simulink model "testFT_sensor"  (Simulink 8.7)
settings: Solver=FixedStepDiscrete  StartTime=0.0  StopTime=inf  FixedStep=ts  RelTol=1e-3
values from neighbouring files (symbols this model uses):
  gazebo_H_base = [Rfoot posFoot; 0 0 0 1]    [initTorqueBalancing.m]    (also in initTorqueBalancingPC.m)
  gazebo_H_chair = [eye(3),[0;0;0.165]; 0 0 0 1]    [initTorqueBalancing.m]    (also in initTorqueBalancingPC.m)
  link2_corr = -9.8    [initTorqueBalancing.m]    (also in initTorqueBalancingPC.m)
undefined symbols (not defined in the file or in its folder): CONFIG, WBT_robotName
libraries: WBToolboxLibrary x13
settings Model: Creator=DanielePucci  LastModifiedBy=gnava
settings DataIOCC: LimitDataPoints=off  SaveFormat=Dataset
settings DebuggingCC: UnderspecifiedInitializationDetection=Simplified  MergeDetectMultiDrivingBlocksExec=error
settings HardwareCC: ProdBitPerPointer=64  ProdLargestAtomicFloat=Float  ProdIntDivRoundTo=Zero  ProdEndianess=LittleEndian  ProdWordSize=64  ProdHWDeviceType=Intel->x86-64 (Windows64)
settings ModelReferenceCC: PropagateSignalLabelsOutOfModel=on
settings ConfigComp: CovModelRefEnable=off

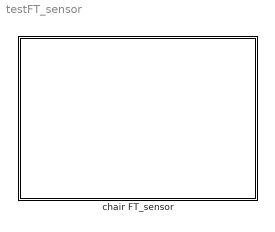
== system testFT_sensor ==
  chair FT_sensor : Subsystem

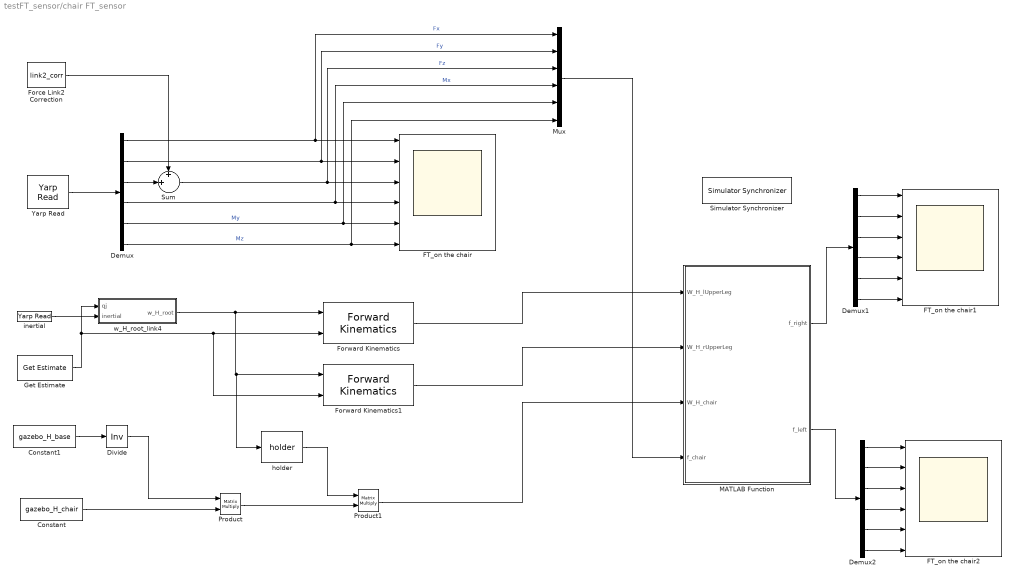
== system testFT_sensor/chair FT_sensor ==
  Constant : Constant  Value=gazebo_H_chair
  Constant1 : Constant  Value=gazebo_H_base
  Demux : Demux  Outputs=6
  Demux1 : Demux  Outputs=6
  Demux2 : Demux  Outputs=6
  Divide : Product  Inputs=/  Multiplication=Matrix(*)
  FT_on the chair : Scope  NumInputPorts=6
  FT_on the chair1 : Scope  NumInputPorts=6
  FT_on the chair2 : Scope  NumInputPorts=6
  Force Link2 Correction : Constant  Value=link2_corr
  Forward Kinematics : WBToolboxLibrary/wholeBodyModel/Kinematics/Forward Kinematics  frameName='l_upper_leg'  robotName=WBT_robotName  localName=WBT_modelName  wbiFile=WBT_wbiFilename  wbiList=WBT_wbiList
  Forward Kinematics1 : WBToolboxLibrary/wholeBodyModel/Kinematics/Forward Kinematics  frameName='r_upper_leg'  robotName=WBT_robotName  localName=WBT_modelName  wbiFile=WBT_wbiFilename  wbiList=WBT_wbiList
  Get Estimate : WBToolboxLibrary/wholeBodyStates/Get Estimate  estimateType=Joints Position  robotName=WBT_robotName  localName=WBT_modelName  wbiFile=WBT_wbiFilename  wbiList=WBT_wbiList
  MATLAB Function : MATLAB Function  TreatAsAtomicUnit=on
  Mux : Mux  Inputs=6
  Product : Product  Multiplication=Matrix(*)
  Product1 : Product  Multiplication=Matrix(*)
  Simulator Synchronizer : WBToolboxLibrary/Utilities/Simulator Synchronizer  period=ts  serverPortName='/clock/rpc'  clientPortName='/WBT_synchronizer/rpc:o'
  Sum : Sum  Inputs=+|+||
  Yarp Read : WBToolboxLibrary/Utilities/Yarp Read  portName=PORTS.WBDT_CHAIR  signalSize=6  blocking=off  timestamp=off  autoconnect=on  errorOnConnection=on
  "holder " : WBToolboxLibrary/Utilities/holder 
  inertial : WBToolboxLibrary/Utilities/Yarp Read  portName=PORTS.IMU  signalSize=12  blocking=off  timestamp=off  autoconnect=on  errorOnConnection=on
  w_H_root_link4 : Subsystem  mask{link_name='l_sole'}
      mask prompts: link_name "link name"
      mask help:
      | This block evaluates the homogeneous transformation between the world and the root link, i.e. ^wH_b. It assumes that the link specified by the variable 'link_name' has a constant position
      | w.r.t. an inertial frame, but it can rotate arbitrarily. This rotation is retrived from the IMU sensor.
      mask Display:
      | str = strrep(link_name, '_','\_');
      | port_label('output',1,['{}^{',str '}H_{root}'],'texmode','on')
      | clear str;
      | 
      | port_label('input',1,'q_j','texmode','on')
      | 
      | port_label('input',2,'inertial','texmode','on')
  wires:
  Demux1/4 -> FT_on the chair1/4
  Constant1/1 -> Divide/1
  MATLAB Function/2(f_left) -> Demux2/1
  MATLAB Function/1(f_right) -> Demux1/1
  Product/1 -> Product1/2
  Demux1/5 -> FT_on the chair1/5
  Demux1/6 -> FT_on the chair1/6
  Demux1/2 -> FT_on the chair1/2
  Forward Kinematics/1 -> MATLAB Function/1(W_H_lUpperLeg)
  "holder "/1 -> Product1/1
  Demux2/4 -> FT_on the chair2/4
  w_H_root_link4/1(w_H_root) -> "holder "/1, Forward Kinematics1/1, Forward Kinematics/1
  Demux1/1 -> FT_on the chair1/1
  Forward Kinematics1/1 -> MATLAB Function/2(W_H_rUpperLeg)
  Mux/1 -> MATLAB Function/4(f_chair)
  Product1/1 -> MATLAB Function/3(W_H_chair)
  Divide/1 -> Product/1
  Constant/1 -> Product/2
  Demux1/3 -> FT_on the chair1/3
  Demux2/2 -> FT_on the chair2/2
  Demux2/5 -> FT_on the chair2/5
  Demux2/3 -> FT_on the chair2/3
  Demux2/6 -> FT_on the chair2/6
  Demux2/1 -> FT_on the chair2/1
  Yarp Read/1 -> Demux/1
  Demux/1 -> FT_on the chair/1, Mux/1  "Fx"
  Demux/2 -> FT_on the chair/2, Mux/2  "Fy"
  Demux/5 -> FT_on the chair/5, Mux/5  "My"
  Demux/4 -> FT_on the chair/4, Mux/4  "Mx"
  Demux/6 -> FT_on the chair/6, Mux/6  "Mz"
  Force Link2 Correction/1 -> Sum/1
  Demux/3 -> Sum/2
  Sum/1 -> FT_on the chair/3, Mux/3  "Fz"
  Get Estimate/1 -> Forward Kinematics1/2, Forward Kinematics/2, w_H_root_link4/1(qj)
  inertial/1 -> w_H_root_link4/2(inertial)

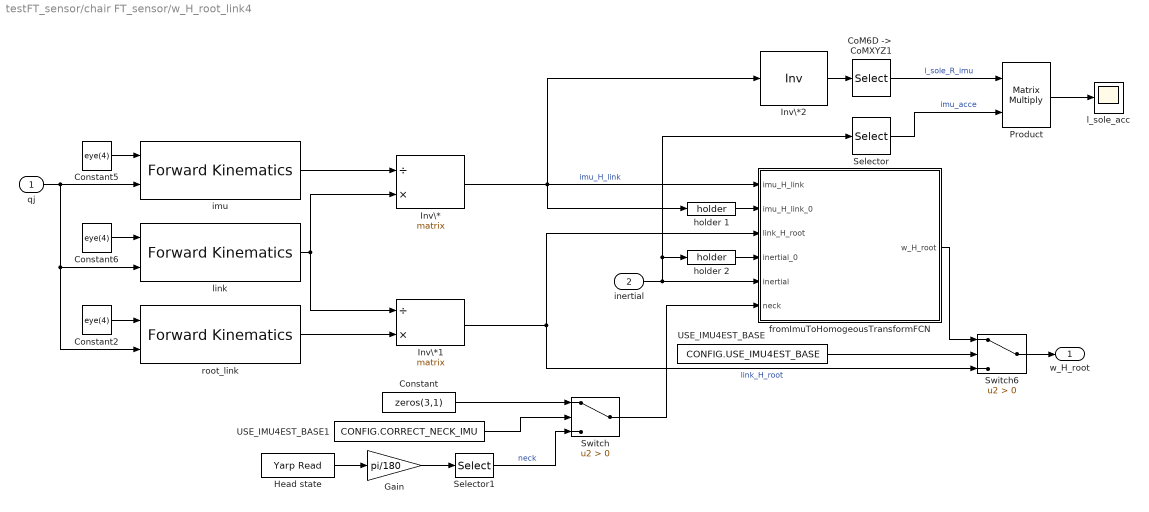
== system testFT_sensor/chair FT_sensor/w_H_root_link4 ==
  qj : Inport
  inertial : Inport  Port=2
  "CoM6D ->  CoMXYZ1" : Selector  NumberOfDimensions=2  InputPortWidth=7  IndexOptions=Index vector (dialog),Index vector (dialog)  Indices=[1 2 3],[1 2 3]  OutputSizes=1,1
  Constant : Constant  Value=zeros(3,1)
  Constant2 : Constant  Value=eye(4)
  Constant5 : Constant  Value=eye(4)
  Constant6 : Constant  Value=eye(4)
  Gain : Gain  Gain=pi/180
  Head state : WBToolboxLibrary/Utilities/Yarp Read  portName=[WBT_robotName, '/head/state:o']  signalSize=6  blocking=off  timestamp=off  autoconnect=on  errorOnConnection=off
  Inv\* : Product  Inputs=/*  Multiplication=Matrix(*)
  Inv\*1 : Product  Inputs=/*  Multiplication=Matrix(*)
  Inv\*2 : Product  Inputs=/  Multiplication=Matrix(*)
  Product : Product  Multiplication=Matrix(*)
  Selector : Selector  InputPortWidth=12  IndexOptions=Index vector (dialog)  Indices=[4 5 6 ]  OutputSizes=1
  Selector1 : Selector  InputPortWidth=6  IndexOptions=Index vector (dialog)  Indices=[1:3]  OutputSizes=1
  Switch : Switch  Criteria=u2 > Threshold
  Switch6 : Switch  Criteria=u2 > Threshold
  USE_IMU4EST_BASE : Constant  Value=CONFIG.USE_IMU4EST_BASE
  USE_IMU4EST_BASE1 : Constant  Value=CONFIG.CORRECT_NECK_IMU
  fromImuToHomogeousTransformFCN : MATLAB Function  TreatAsAtomicUnit=on
  holder 1 : WBToolboxLibrary/Utilities/holder 
  holder 2 : WBToolboxLibrary/Utilities/holder 
  imu : WBToolboxLibrary/wholeBodyModel/Kinematics/Forward Kinematics  frameName='imu_frame'  robotName=WBT_robotName  localName=WBT_modelName  wbiFile=WBT_wbiFilename  wbiList=WBT_wbiList
  l_sole_acc : Scope
  link : WBToolboxLibrary/wholeBodyModel/Kinematics/Forward Kinematics  frameName=link_name  robotName=WBT_robotName  localName=WBT_modelName  wbiFile=WBT_wbiFilename  wbiList=WBT_wbiList
  root_link : WBToolboxLibrary/wholeBodyModel/Kinematics/Forward Kinematics  frameName='root_link'  robotName=WBT_robotName  localName=WBT_modelName  wbiFile=WBT_wbiFilename  wbiList=WBT_wbiList
  w_H_root : Outport
  wires:
  Constant5/1 -> imu/1
  Inv\*/1 -> Inv\*2/1, holder 1/1, fromImuToHomogeousTransformFCN/1(imu_H_link)  "imu_H_link"
  imu/1 -> Inv\*/1
  Constant6/1 -> link/1
  Inv\*1/1 -> Switch6/3, fromImuToHomogeousTransformFCN/3(link_H_root)  "link_H_root"
  link/1 -> Inv\*/2, Inv\*1/1
  inertial/1 -> Selector/1, holder 2/1, fromImuToHomogeousTransformFCN/5(inertial)
  Switch6/1 -> w_H_root/1
  USE_IMU4EST_BASE/1 -> Switch6/2
  fromImuToHomogeousTransformFCN/1(w_H_root) -> Switch6/1
  Constant2/1 -> root_link/1
  qj/1 -> root_link/2, link/2, imu/2
  root_link/1 -> Inv\*1/2
  holder 1/1 -> fromImuToHomogeousTransformFCN/2(imu_H_link_0)
  holder 2/1 -> fromImuToHomogeousTransformFCN/4(inertial_0)
  Inv\*2/1 -> "CoM6D ->  CoMXYZ1"/1
  "CoM6D ->  CoMXYZ1"/1 -> Product/1  "l_sole_R_imu"
  Selector/1 -> Product/2  "imu_acce"
  Product/1 -> l_sole_acc/1
  Head state/1 -> Gain/1
  Selector1/1 -> Switch/3  "neck"
  Constant/1 -> Switch/1
  USE_IMU4EST_BASE1/1 -> Switch/2
  Switch/1 -> fromImuToHomogeousTransformFCN/6(neck)
  Gain/1 -> Selector1/1

== matlab function chair FT_sensor/MATLAB Function ==
  data: W_H_lUpperLeg input double; f_right output double; W_H_rUpperLeg input double; W_H_chair input double; f_chair input double; f_left output double
function [f_right,f_left] = fcn(W_H_lUpperLeg,W_H_rUpperLeg,W_H_chair,f_chair)
%#codegen
w_R_lup   = W_H_lUpperLeg(1:3,1:3);
w_R_rup   = W_H_rUpperLeg(1:3,1:3);
w_R_chair = W_H_chair(1:3,1:3);

w_pos_lup   = W_H_lUpperLeg(1:3,4);
w_pos_rup   = W_H_rUpperLeg(1:3,4);
w_pos_chair = W_H_chair(1:3,4);

dist_chair_lup = w_pos_lup-w_pos_chair;
dist_chair_rup = w_pos_rup-w_pos_chair;

lup_R_chair    = transpose(w_R_lup)*w_R_chair;
rup_R_chair    = transpose(w_R_rup)*w_R_chair;

f_chair_half   = f_chair./2;

lup_X_chair    = [lup_R_chair -lup_R_chair*skew(dist_chair_lup);
                  zeros(3)     lup_R_chair];

rup_X_chair    = [rup_R_chair -rup_R_chair*skew(dist_chair_rup);
                  zeros(3)     rup_R_chair];  
              
f_right = rup_X_chair*f_chair_half;
f_left  = lup_X_chair*f_chair_half;

end

== matlab function chair FT_sensor/w_H_root_link4/fromImuToHomogeousTransformFCN ==
  data: imu_H_link input double; imu_H_link_0 input double; link_H_root input double; inertial_0 input double; inertial input double; neck input double; w_H_root output double; CONFIG parameter double
function w_H_root = fromBaseToWorldWithImuFCN(imu_H_link,imu_H_link_0,link_H_root,inertial_0,inertial,neck,CONFIG)
%#codegen
w_H_root = fromBaseToWorldWithImu(imu_H_link,imu_H_link_0,link_H_root,inertial_0,inertial,neck,CONFIG);
